simulink model "M_FLCC"  (R2022a)
settings: Solver=ode4  StartTime=0.0  StopTime=100  FixedStep=0.01  RelTol=1e-3
PreLoadFcn:
  | load('BUS_STRUCTURE_FLCC.mat');
InitFcn:
  | load('BUS_STRUCTURE_FLCC.mat');
undefined symbols (not defined in the file or in its folder): f16data
libraries: sharedtransform x6, simulink_extras x4, aerolibatmos2 x1
(part 1 of 2)
settings Model: Creator=ASCL  LastModifiedBy=ASCL
settings DataIOCC: SaveOutput=off  SignalLogging=off  DSMLogging=off  SaveTime=off  ReturnWorkspaceOutputs=off
settings OptimizationCC: BlockReduction=off  DefaultParameterBehavior=Inlined  UseDivisionForNetSlopeComputation=on  GainParamInheritBuiltInType=on  UseFloatMulNetSlope=on  ExpressionFolding=off  PassReuseOutputArgsAs=Individual arguments  ZeroExternalMemoryAtStartup=off  ZeroInternalMemoryAtStartup=off  EfficientFloat2IntCast=on  LifeSpan=inf  OptimizeBlockOrder=speed  DifferentSizesBufferReuse=on  EfficientTunableParamExpr=on
settings DebuggingCC: SignalInfNanChecking=warning  ReadBeforeWriteMsg=EnableAllAsError  WriteAfterWriteMsg=EnableAllAsError  WriteAfterReadMsg=EnableAllAsError  IntegerOverflowMsg=error  ParameterTunabilityLossMsg=error  UniqueDataStoreMsg=error  AssertControl=DisableAll  NonBusSignalsTreatedAsBus=error  SFInvalidInputDataAccessInChartInitDiag=error  SFTransitionOutsideNaturalParentDiag=error  SFUnreachableExecutionPathDiag=error  SFUndirectedBroadcastEventsDiag=error  IntegerSaturationMsg=error
settings HardwareCC: ProdBitPerPointer=32  ProdBitPerSizeT=32  ProdBitPerPtrDiffT=32  ProdLargestAtomicInteger=Long  ProdLargestAtomicFloat=Double  ProdEndianess=BigEndian  ProdWordSize=32  ProdLongLongMode=on  ProdHWDeviceType=Freescale->MPC83xx
settings ModelReferenceCC: ModelReferenceNumInstancesAllowed=Single
settings SFSimCC: SimCustomHeaderCode="#include \"MAP.h\""  SimUserSources=MAP.c  SimUserLibraries=WS2_32.LIB  CompileTimeRecursionLimit=0  EnableRuntimeRecursion=off  MATLABDynamicMemAlloc=off
settings RTWCC: SystemTargetFile=ert.tlc  TemplateMakefile=ert_default_tmf  GenerateReport=on  RTWUseSimCustomCode=on  CustomHeaderCode="#include \"MAP.h\""  CustomSource=MAP.c  CustomLibrary=WS2_32.LIB  BuildConfiguration=Faster Runs  IncludeHyperlinkInReport=on  LaunchReport=on  GenerateTraceInfo=on  GenerateTraceReport=on  GenerateTraceReportSl=on  GenerateTraceReportSf=on  GenerateTraceReportEml=on
settings CodeAppCC: ForceParamTrailComments=on  IgnoreCustomStorageClasses=off  OperatorAnnotations=on  SimulinkDataObjDesc=on  SFDataObjDesc=on  MATLABFcnDesc=on  InsertBlockDesc=on  StateflowObjectComments=on  MATLABSourceComments=on  EnableCustomComments=on  InlinedPrmAccess=Macros  ReqsInCode=on
settings ERTTargetCC: TargetLangStandard=C99 (ISO)  UtilityFuncGeneration=Shared location  GenerateSampleERTMain=on  IncludeMdlTerminateFcn=off  CombineSignalStateStructs=on  SupportAbsoluteTime=off  SupportNonFinite=off  SupportVariableSizeSignals=on  ParenthesesLevel=Standards  CastingMode=Standards  GenerateSharedConstants=off  InlinedParameterPlacement=NonHierarchical  ERTCustomFileTemplate=example_file_process.tlc  RateTransitionBlockCode=Function  PreserveIfCondition=on  ConvertIfToSwitch=off  EnableSignedLeftShifts=off  EnableSignedRightShifts=off

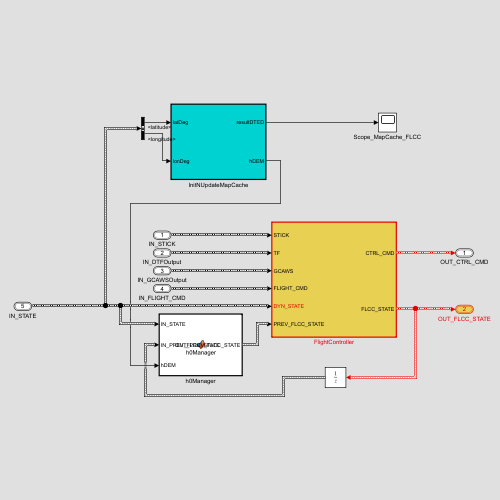
[thumbnail: Simulink's stored preview of the top-level diagram]
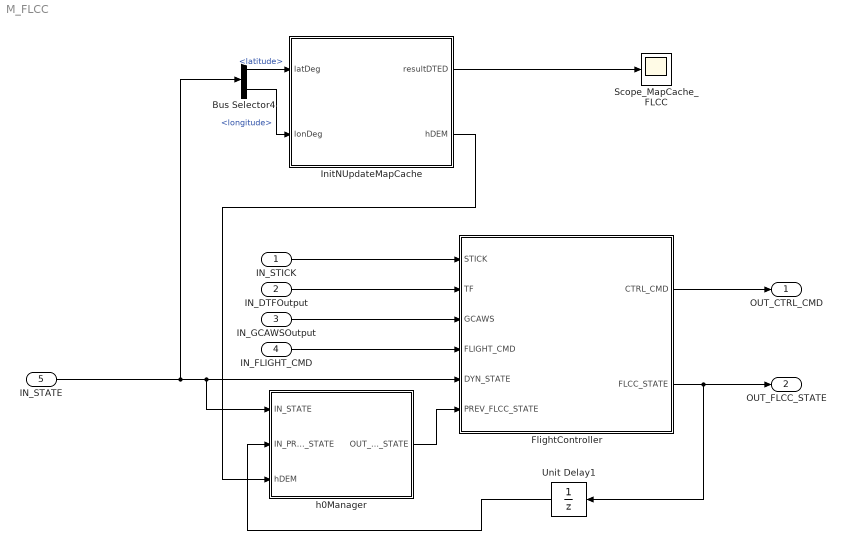
== system M_FLCC ==
  IN_STICK : Inport  OutDataTypeStr=Bus: BUS_FLCC_STICK  Interpolate=off  BusOutputAsStruct=on
  IN_DTFOutput : Inport  Port=2  OutDataTypeStr=Bus: DTFOutput  Interpolate=off  BusOutputAsStruct=on
  IN_GCAWSOutput : Inport  Port=3  OutDataTypeStr=Bus: GCAWSOutput  Interpolate=off  BusOutputAsStruct=on
  IN_FLIGHT_CMD : Inport  Port=4  OutDataTypeStr=Bus: BUS_FLCC_FLIGHT_CMD  Interpolate=off  BusOutputAsStruct=on
  IN_STATE : Inport  Port=5  OutDataTypeStr=Bus: BUS_DYN_STATE  Interpolate=off  BusOutputAsStruct=on
  Bus Selector4 : BusSelector  OutputSignals=latitude,longitude
  FlightController : Subsystem  TreatAsAtomicUnit=on
  InitNUpdateMapCache : Subsystem  TreatAsAtomicUnit=on
  Scope_MapCache_FLCC : Scope
  Unit Delay1 : UnitDelay  SampleTime=0.01  HasFrameUpgradeWarning=on
  h0Manager : MATLAB Function  TreatAsAtomicUnit=on
  OUT_CTRL_CMD : Outport  OutDataTypeStr=Bus: BUS_FLCC_CTRL_CMD  VectorParamsAs1DForOutWhenUnconnected=off  BusOutputAsStruct=on
  OUT_FLCC_STATE : Outport  Port=2  OutDataTypeStr=Bus: BUS_FLCC_AP_STATE  VectorParamsAs1DForOutWhenUnconnected=off  BusOutputAsStruct=on
  wires:
  FlightController/1(CTRL_CMD) -> OUT_CTRL_CMD/1
  IN_STICK/1 -> FlightController/1(STICK)
  IN_STATE/1 -> Bus Selector4/1, h0Manager/1(IN_STATE), FlightController/5(DYN_STATE)
  IN_DTFOutput/1 -> FlightController/2(TF)
  FlightController/2(FLCC_STATE) -> OUT_FLCC_STATE/1, Unit Delay1/1
  IN_GCAWSOutput/1 -> FlightController/3(GCAWS)
  Unit Delay1/1 -> h0Manager/2(IN_PREV_FLCC_STATE)
  Bus Selector4/1 -> InitNUpdateMapCache/1(latDeg)  "<latitude>"
  Bus Selector4/2 -> InitNUpdateMapCache/2(lonDeg)  "<longitude>"
  InitNUpdateMapCache/1(resultDTED) -> Scope_MapCache_FLCC/1
  h0Manager/1(OUT_PREV_FLCC_STATE) -> FlightController/6(PREV_FLCC_STATE)
  InitNUpdateMapCache/2(hDEM) -> h0Manager/3(hDEM)
  IN_FLIGHT_CMD/1 -> FlightController/4(FLIGHT_CMD)

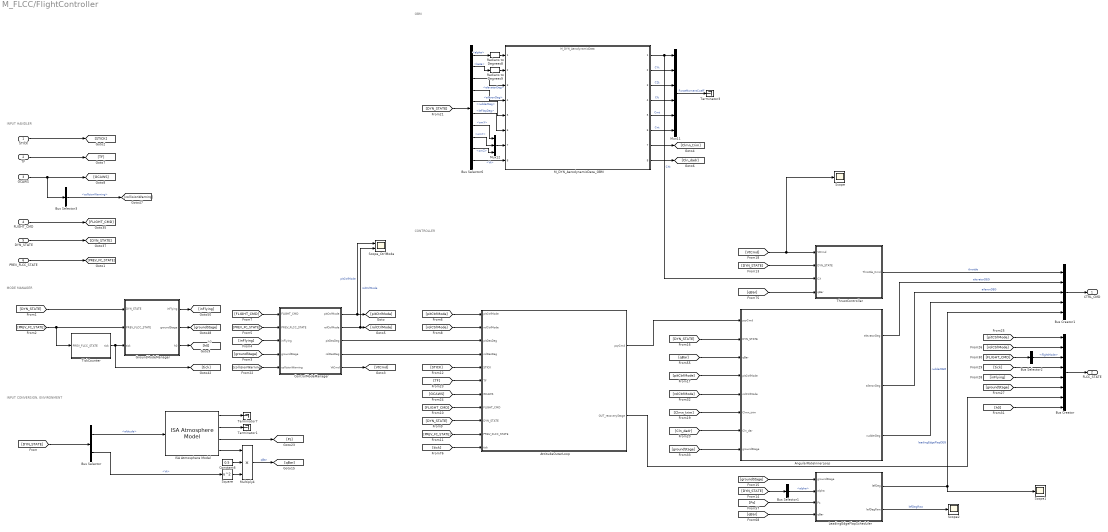
== system M_FLCC/FlightController ==
  note: h0
  note: OBM
  note: CONTROLLER
  note: MODE MANAGER
  note: INPUT CONVERSION, ENVIRONMENT
  note: INPUT HANDLER
  STICK : Inport  OutDataTypeStr=Bus: BUS_FLCC_STICK
  TF : Inport  Port=2  OutDataTypeStr=Bus: DTFOutput
  GCAWS : Inport  Port=3  OutDataTypeStr=Bus: GCAWSOutput
  FLIGHT_CMD : Inport  Port=4  OutDataTypeStr=Bus: BUS_FLCC_FLIGHT_CMD
  DYN_STATE : Inport  Port=5  OutDataTypeStr=Bus: BUS_DYN_STATE
  PREV_FLCC_STATE : Inport  Port=6  OutDataTypeStr=Bus: BUS_FLCC_AP_STATE
  AngularRateInnerLoop : Subsystem
  AttitudeOuterLoop : Subsystem
  Bus Creator : BusCreator  Inputs=8  OutDataTypeStr=Bus: BUS_FLCC_AP_STATE  NonVirtualBus=on
      settings: InheritFromInputs=off
  Bus Creator1 : BusCreator  Inputs=5  OutDataTypeStr=Bus: BUS_FLCC_CTRL_CMD  NonVirtualBus=on
      settings: InheritFromInputs=off
  Bus Selector : BusSelector  OutputSignals=altitude,Vt
  Bus Selector1 : BusSelector  OutputSignals=alpha
  Bus Selector2 : BusSelector  OutputSignals=flightMode
  Bus Selector3 : BusSelector  OutputSignals=collisionWarning
  Bus Selector6 : BusSelector  OutputSignals=alpha,beta,elevatorDeg,aileronDeg,rudderDeg,leFlapDeg,omX,omY,omZ,Vt
  Constant6 : Constant  Value=0.5
  ControlModeManager : MATLAB Function  TreatAsAtomicUnit=on
  GroundModeManager : MATLAB Function  TreatAsAtomicUnit=on
  ISA Atmosphere Model : aerolibatmos2/ISA Atmosphere Model  custom=off  g=9.80665  gamma=1.4  R=287.0531  L=0.0065  h_trop=11000  h_strat=20000  rho0=1.225  P0=101325  T0=288.15  h0=0
  LeadingEdgeFlapScheduler : MATLAB Function  TreatAsAtomicUnit=on
  M_DYN_AerodynamicData_OBM : ModelReference  ModelNameDialog=M_DYN_AerodynamicData.slx  SimulationMode=Normal  ModelReferenceVersion=1.97
  Multiply4 : Product  Inputs=3
  Mux11 : Mux  Inputs=6
  Mux12 : Mux  Inputs=3
  Radians to Degrees8 : simulink_extras/Transformations/Radians to Degrees
  Radians to Degrees9 : simulink_extras/Transformations/Radians to Degrees
  Scope : Scope
  Scope1 : Scope
  Scope2 : Scope
  Scope_CtrlMode : Scope  NumInputPorts=2
  Square : Math  Operator=square  SignedPower=on
  Terminator1 : Terminator
  Terminator3 : Terminator
  Terminator7 : Terminator
  ThrustController : Subsystem
  TickCounter : MATLAB Function  TreatAsAtomicUnit=on
  CTRL_CMD : Outport  OutDataTypeStr=Bus: BUS_FLCC_CTRL_CMD  VectorParamsAs1DForOutWhenUnconnected=off
  FLCC_STATE : Outport  Port=2  OutDataTypeStr=Bus: BUS_FLCC_AP_STATE  VectorParamsAs1DForOutWhenUnconnected=off
  wires:
  DYN_STATE/1 -> [DYN_STATE]
  ISA Atmosphere Model/1 -> Terminator7/1
  ISA Atmosphere Model/2 -> Terminator1/1
  ISA Atmosphere Model/3 -> [Ps]
  ISA Atmosphere Model/4 -> Multiply4/1
  Constant6/1 -> Multiply4/2
  Square/1 -> Multiply4/3
  Multiply4/1 -> [qBar]  "qBar"
  LeadingEdgeFlapScheduler/1(lefDeg) -> Scope1/1, Bus Creator1/5  "leadingEdgeFlapDEG"
  Bus Creator/1 -> FLCC_STATE/1
  [pitCtrlMode] -> Bus Creator/1
  [rolCtrlMode] -> Bus Creator/2
  Bus Selector3/1 -> [collisionWarning]  "<collisionWarning>"
  TickCounter/1(tick) -> [tick], GroundModeManager/3(tick)
  GroundModeManager/1(inFlying) -> [inFlying]
  ControlModeManager/2(rolCtrlMode) -> Scope_CtrlMode/2, [rolCtrlMode]  "rolCtrlMode"
  ControlModeManager/1(pitCtrlMode) -> Scope_CtrlMode/1, [pitCtrlMode]  "pitCtrlMode"
  [Ps] -> LeadingEdgeFlapScheduler/3(Ps)
  [qBar] -> LeadingEdgeFlapScheduler/4(qBar)
  GroundModeManager/2(groundStage) -> [groundStage]
  STICK/1 -> [STICK]
  AttitudeOuterLoop/1(pqrCmd) -> AngularRateInnerLoop/1(pqrCmd)
  M_DYN_AerodynamicData_OBM/6 -> Mux11/6  "Cnt"
  M_DYN_AerodynamicData_OBM/5 -> Mux11/5  "Cmt"
  M_DYN_AerodynamicData_OBM/4 -> Mux11/4  "Clt"
  M_DYN_AerodynamicData_OBM/2 -> Mux11/2  "CYt"
  M_DYN_AerodynamicData_OBM/1 -> Mux11/1, ThrustController/3(CX)  "CXt"
  M_DYN_AerodynamicData_OBM/3 -> Mux11/3  "CZt"
  Mux11/1 -> Terminator3/1  "ForceMomentCoeff"
  [qBar] -> AngularRateInnerLoop/3(qBar)
  [qBar] -> ThrustController/4(qBar)
  ThrustController/1(Throttle_Cmd) -> Bus Creator1/1  "throttle"
  Bus Selector6/10 -> M_DYN_AerodynamicData_OBM/8  "<Vt>"
  Bus Selector6/1 -> Radians to Degrees8/1  "<alpha>"
  Bus Selector6/2 -> Radians to Degrees9/1  "<beta>"
  Radians to Degrees8/1 -> M_DYN_AerodynamicData_OBM/1
  Radians to Degrees9/1 -> M_DYN_AerodynamicData_OBM/2
  Bus Selector6/3 -> M_DYN_AerodynamicData_OBM/3  "<elevatorDeg>"
  Bus Selector6/4 -> M_DYN_AerodynamicData_OBM/4  "<aileronDeg>"
  Bus Selector6/5 -> M_DYN_AerodynamicData_OBM/5  "<rudderDeg>"
  Bus Selector6/6 -> M_DYN_AerodynamicData_OBM/6  "<leFlapDeg>"
  Mux12/1 -> M_DYN_AerodynamicData_OBM/7
  Bus Selector6/9 -> Mux12/3  "<omZ>"
  Bus Selector6/8 -> Mux12/2  "<omY>"
  Bus Selector6/7 -> Mux12/1  "<omX>"
  [tick] -> AttitudeOuterLoop/11(tick)
  ControlModeManager/3(pitDesDeg) -> AttitudeOuterLoop/3(pitDesDeg)
  ControlModeManager/4(rolDesDeg) -> AttitudeOuterLoop/4(rolDesDeg)
  [DYN_STATE] -> Bus Selector/1
  [DYN_STATE] -> GroundModeManager/1(DYN_STATE)
  PREV_FLCC_STATE/1 -> [PREV_FC_STATE]
  [PREV_FC_STATE] -> TickCounter/1(PREV_FLCC_STATE), GroundModeManager/2(PREV_FLCC_STATE)
  [groundStage] -> ControlModeManager/4(groundStage)
  [inFlying] -> ControlModeManager/3(inFlying)
  [PREV_FC_STATE] -> ControlModeManager/2(PREV_FLCC_STATE)
  [FLIGHT_CMD] -> ControlModeManager/1(FLIGHT_CMD)
  Bus Selector/1 -> ISA Atmosphere Model/1  "<altitude>"
  Bus Selector/2 -> Square/1  "<Vt>"
  [DYN_STATE] -> AttitudeOuterLoop/9(DYN_STATE)
  [FLIGHT_CMD] -> AttitudeOuterLoop/8(FLIGHT_CMD)
  [PREV_FC_STATE] -> AttitudeOuterLoop/10(PREV_FLCC_STATE)
  [STICK] -> AttitudeOuterLoop/5(STICK)
  [DYN_STATE] -> ThrustController/2(DYN_STATE)
  [DYN_STATE] -> Bus Selector1/1
  Bus Selector1/1 -> LeadingEdgeFlapScheduler/2(alpha)  "<alpha>"
  [groundStage] -> LeadingEdgeFlapScheduler/1(groundStage)
  [DYN_STATE] -> AngularRateInnerLoop/2(DYN_STATE)
  Bus Creator1/1 -> CTRL_CMD/1
  AngularRateInnerLoop/1(elevatorDeg) -> Bus Creator1/2  "elevatorDEG"
  AngularRateInnerLoop/2(aileronDeg) -> Bus Creator1/3  "aileronDEG"
  AngularRateInnerLoop/3(rudderDeg) -> Bus Creator1/4  "rudderDEG"
  ControlModeManager/5(VtCmd) -> [VtCmd]
  [VtCmd] -> Scope/1, ThrustController/1(VtCmd)
  M_DYN_AerodynamicData_OBM/8 -> [Cln_dadr]
  M_DYN_AerodynamicData_OBM/7 -> [Clmn_trim]
  [Clmn_trim] -> AngularRateInnerLoop/6(Clmn_trim)
  [Cln_dadr] -> AngularRateInnerLoop/7(Cln_dar)
  [DYN_STATE] -> Bus Selector6/1
  [collisionWarning] -> ControlModeManager/5(collisionWarning)
  GCAWS/1 -> Bus Selector3/1, [GCAWS]
  TF/1 -> [TF]
  [GCAWS] -> AttitudeOuterLoop/7(GCAWS)
  [TF] -> AttitudeOuterLoop/6(TF)
  [rolCtrlMode] -> AttitudeOuterLoop/2(rolCtrlMode)
  [pitCtrlMode] -> AttitudeOuterLoop/1(pitCtrlMode)
  [groundStage] -> Bus Creator/6
  [inFlying] -> Bus Creator/5
  [tick] -> Bus Creator/4
  AttitudeOuterLoop/2(OUT_recoveryStage) -> Bus Creator/7
  [FLIGHT_CMD] -> Bus Selector2/1
  Bus Selector2/1 -> Bus Creator/3  "<flightMode>"
  GroundModeManager/3(h0) -> [h0]
  [h0] -> Bus Creator/8
  [pitCtrlMode] -> AngularRateInnerLoop/4(pitCtrlMode)
  [rolCtrlMode] -> AngularRateInnerLoop/5(rolCtrlMode)
  [groundStage] -> AngularRateInnerLoop/8(groundStage)
  LeadingEdgeFlapScheduler/2(lefDegRaw) -> Scope2/1  "lefDegRaw"
  FLIGHT_CMD/1 -> [FLIGHT_CMD]

== system M_FLCC/InitNUpdateMapCache ==
  latDeg : Inport  OutDataTypeStr=double
  lonDeg : Inport  Port=2  OutDataTypeStr=double
  If : If  NumInputs=2  IfExpression=(u1 == 0)  ShowElse=off
  InitializeMAP : MATLAB Function  TreatAsAtomicUnit=on  SystemSampleTime=0.01
  UpdateCache : Subsystem  TreatAsAtomicUnit=on
  resultDTED : Outport  VectorParamsAs1DForOutWhenUnconnected=off
  hDEM : Outport  Port=2
  wires:
  lonDeg/1 -> InitializeMAP/2(lonDeg), UpdateCache/2(lon)
  UpdateCache/1(result) -> resultDTED/1
  InitializeMAP/1(successDTED) -> If/1
  latDeg/1 -> InitializeMAP/1(latDeg), UpdateCache/1(lat)
  InitializeMAP/2(successDVOF) -> If/2
  If/1 -> UpdateCache/Action
  UpdateCache/2(hDEM) -> hDEM/1

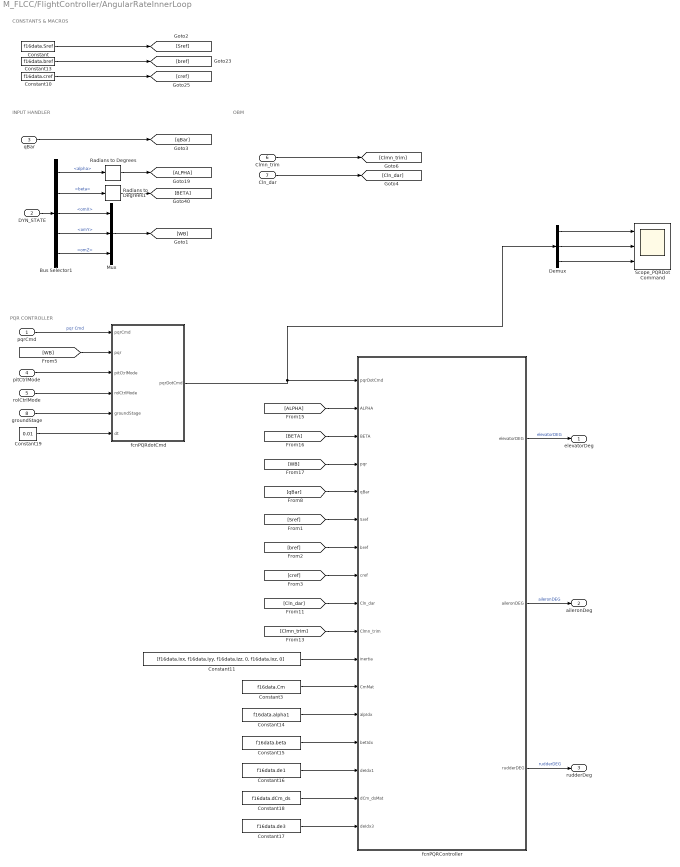
== system M_FLCC/FlightController/AngularRateInnerLoop ==
  note: PQR CONTROLLER
  note: INPUT HANDLER
  note: OBM
  note: CONSTANTS & MACROS
  pqrCmd : Inport
  DYN_STATE : Inport  Port=2
  qBar : Inport  Port=3
  pitCtrlMode : Inport  Port=4
  rolCtrlMode : Inport  Port=5
  Clmn_trim : Inport  Port=6
  Cln_dar : Inport  Port=7
  groundStage : Inport  Port=8
  Bus Selector1 : BusSelector  OutputSignals=alpha,beta,omX,omY,omZ
  Constant : Constant  Value=f16data.Sref
  Constant10 : Constant  Value=f16data.cref
  Constant11 : Constant  Value=[f16data.Ixx, f16data.Iyy, f16data.Izz, 0, f16data.Ixz, 0]
  Constant13 : Constant  Value=f16data.bref
  Constant14 : Constant  Value=f16data.alpha1
  Constant15 : Constant  Value=f16data.beta
  Constant16 : Constant  Value=f16data.de1
  Constant17 : Constant  Value=f16data.de3
  Constant18 : Constant  Value=f16data.dCm_ds
  Constant19 : Constant  Value=0.01
  Constant3 : Constant  Value=f16data.Cm
  Demux : Demux  Outputs=3
  Mux : Mux  Inputs=3
  Radians to Degrees : simulink_extras/Transformations/Radians to Degrees
  Radians to Degrees1 : simulink_extras/Transformations/Radians to Degrees
  Scope_PQRDot Command : Scope  NumInputPorts=3
  fcnPQRController : MATLAB Function  TreatAsAtomicUnit=on
  fcnPQRdotCmd : MATLAB Function  TreatAsAtomicUnit=on  SystemSampleTime=0.01
  elevatorDeg : Outport
  aileronDeg : Outport  Port=2
  rudderDeg : Outport  Port=3
  wires:
  Bus Selector1/1 -> Radians to Degrees/1  "<alpha>"
  Mux/1 -> [WB]
  Bus Selector1/2 -> Radians to Degrees1/1  "<beta>"
  [WB] -> fcnPQRdotCmd/2(pqr)
  pqrCmd/1 -> fcnPQRdotCmd/1(pqrCmd)  "pqr Cmd"
  Constant11/1 -> fcnPQRController/11(inertia)
  [qBar] -> fcnPQRController/5(qBar)
  qBar/1 -> [qBar]
  [Sref] -> fcnPQRController/6(Sref)
  [bref] -> fcnPQRController/7(bref)
  [cref] -> fcnPQRController/8(cref)
  [Cln_dar] -> fcnPQRController/9(Cln_dar)
  Constant3/1 -> fcnPQRController/12(CmMat)
  Constant14/1 -> fcnPQRController/13(alpIdx)
  Constant15/1 -> fcnPQRController/14(betIdx)
  Constant16/1 -> fcnPQRController/15(deIdx1)
  Constant18/1 -> fcnPQRController/16(dCm_dsMat)
  Constant17/1 -> fcnPQRController/17(deIdx3)
  [ALPHA] -> fcnPQRController/2(ALPHA)
  [BETA] -> fcnPQRController/3(BETA)
  fcnPQRController/1(elevatorDEG) -> elevatorDeg/1  "elevatorDEG"
  fcnPQRController/3(rudderDEG) -> rudderDeg/1  "rudderDEG"
  [WB] -> fcnPQRController/4(pqr)
  [Clmn_trim] -> fcnPQRController/10(Clmn_trim)
  Constant19/1 -> fcnPQRdotCmd/6(dt)
  Clmn_trim/1 -> [Clmn_trim]
  Cln_dar/1 -> [Cln_dar]
  Constant/1 -> [Sref]
  Constant10/1 -> [cref]
  Constant13/1 -> [bref]
  fcnPQRdotCmd/1(pqrDotCmd) -> Demux/1, fcnPQRController/1(pqrDotCmd)
  DYN_STATE/1 -> Bus Selector1/1
  Bus Selector1/3 -> Mux/1  "<omX>"
  Bus Selector1/4 -> Mux/2  "<omY>"
  Bus Selector1/5 -> Mux/3  "<omZ>"
  Radians to Degrees/1 -> [ALPHA]
  Radians to Degrees1/1 -> [BETA]
  fcnPQRController/2(aileronDEG) -> aileronDeg/1  "aileronDEG"
  Demux/3 -> Scope_PQRDot Command/3
  Demux/1 -> Scope_PQRDot Command/1
  Demux/2 -> Scope_PQRDot Command/2
  pitCtrlMode/1 -> fcnPQRdotCmd/3(pitCtrlMode)
  rolCtrlMode/1 -> fcnPQRdotCmd/4(rolCtrlMode)
  groundStage/1 -> fcnPQRdotCmd/5(groundStage)

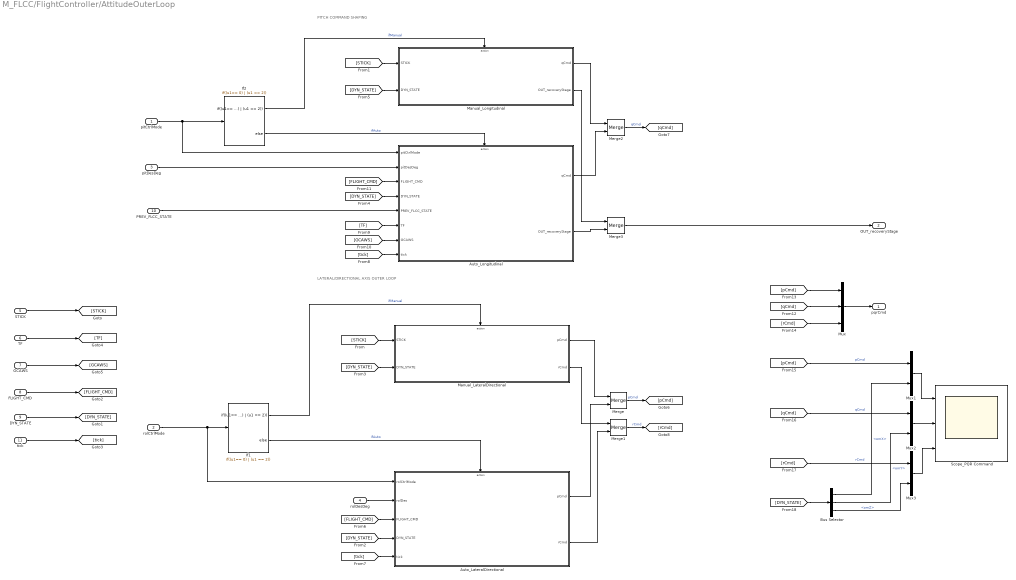
== system M_FLCC/FlightController/AttitudeOuterLoop ==
  note: PITCH COMMAND SHAPING
  note: LATERAL/DIRECTIONAL AXIS OUTER LOOP
  pitCtrlMode : Inport
  rolCtrlMode : Inport  Port=2
  pitDesDeg : Inport  Port=3
  rolDesDeg : Inport  Port=4
  STICK : Inport  Port=5
  TF : Inport  Port=6
  GCAWS : Inport  Port=7
  FLIGHT_CMD : Inport  Port=8
  DYN_STATE : Inport  Port=9
  PREV_FLCC_STATE : Inport  Port=10
  tick : Inport  Port=11
  Auto_LateralDirectional : Subsystem  TreatAsAtomicUnit=on
  Auto_Longitudinal : Subsystem  TreatAsAtomicUnit=on
  Bus Selector : BusSelector  OutputSignals=omX,omY,omZ
  If1 : If  IfExpression=(u1== 0) | (u1 == 2)
  If2 : If  IfExpression=(u1== 0) | (u1 == 2)
  Manual_LateralDirectional : Subsystem  TreatAsAtomicUnit=on
  Manual_Longitudinal : Subsystem  TreatAsAtomicUnit=on
  Merge{,1..3} (4 alike) : Merge
  Mux : Mux  Inputs=3
  Mux1 : Mux  Inputs=2
  Mux2 : Mux  Inputs=2
  Mux3 : Mux  Inputs=2
  Scope_PQR Command : Scope  NumInputPorts=3
  pqrCmd : Outport
  OUT_recoveryStage : Outport  Port=2
  wires:
  rolDesDeg/1 -> Auto_LateralDirectional/2(rolDes)
  rolCtrlMode/1 -> Auto_LateralDirectional/1(rolCtrlMode), If1/1
  If1/1 -> Manual_LateralDirectional/Action  "ifManual"
  If1/2 -> Auto_LateralDirectional/Action  "ifAuto"
  Manual_LateralDirectional/1(pCmd) -> Merge/1
  Auto_LateralDirectional/1(pCmd) -> Merge/2
  Manual_LateralDirectional/2(rCmd) -> Merge1/1
  Auto_LateralDirectional/2(rCmd) -> Merge1/2
  Mux/1 -> pqrCmd/1
  Merge/1 -> [pCmd]  "pCmd"
  Merge1/1 -> [rCmd]  "rCmd"
  pitCtrlMode/1 -> Auto_Longitudinal/1(pitCtrlMode), If2/1
  If2/1 -> Manual_Longitudinal/Action  "ifManual"
  Manual_Longitudinal/1(qCmd) -> Merge2/1
  Merge2/1 -> [qCmd]  "qCmd"
  Auto_Longitudinal/1(qCmd) -> Merge2/2
  pitDesDeg/1 -> Auto_Longitudinal/2(pitDesDeg)
  If2/2 -> Auto_Longitudinal/Action  "ifAuto"
  PREV_FLCC_STATE/1 -> Auto_Longitudinal/5(PREV_FLCC_STATE)
  STICK/1 -> [STICK]
  [STICK] -> Manual_LateralDirectional/1(STICK)
  [STICK] -> Manual_Longitudinal/1(STICK)
  DYN_STATE/1 -> [DYN_STATE]
  [DYN_STATE] -> Auto_LateralDirectional/4(DYN_STATE)
  [DYN_STATE] -> Auto_Longitudinal/4(DYN_STATE)
  [DYN_STATE] -> Manual_Longitudinal/2(DYN_STATE)
  [DYN_STATE] -> Manual_LateralDirectional/2(DYN_STATE)
  FLIGHT_CMD/1 -> [FLIGHT_CMD]
  [FLIGHT_CMD] -> Auto_LateralDirectional/3(FLIGHT_CMD)
  [tick] -> Auto_LateralDirectional/5(tick)
  [tick] -> Auto_Longitudinal/8(tick)
  tick/1 -> [tick]
  TF/1 -> [TF]
  GCAWS/1 -> [GCAWS]
  [TF] -> Auto_Longitudinal/6(TF)
  [GCAWS] -> Auto_Longitudinal/7(GCAWS)
  [FLIGHT_CMD] -> Auto_Longitudinal/3(FLIGHT_CMD)
  Auto_Longitudinal/2(OUT_recoveryStage) -> Merge3/2
  Manual_Longitudinal/2(OUT_recoveryStage) -> Merge3/1
  Merge3/1 -> OUT_recoveryStage/1
  Mux1/1 -> Scope_PQR Command/1
  [qCmd] -> Mux/2
  [pCmd] -> Mux/1
  [rCmd] -> Mux/3
  Mux2/1 -> Scope_PQR Command/2
  Mux3/1 -> Scope_PQR Command/3
  [pCmd] -> Mux1/1  "pCmd"
  [qCmd] -> Mux2/1  "qCmd"
  [rCmd] -> Mux3/1  "rCmd"
  [DYN_STATE] -> Bus Selector/1
  Bus Selector/1 -> Mux1/2  "<omX>"
  Bus Selector/2 -> Mux2/2  "<omY>"
  Bus Selector/3 -> Mux3/2  "<omZ>"

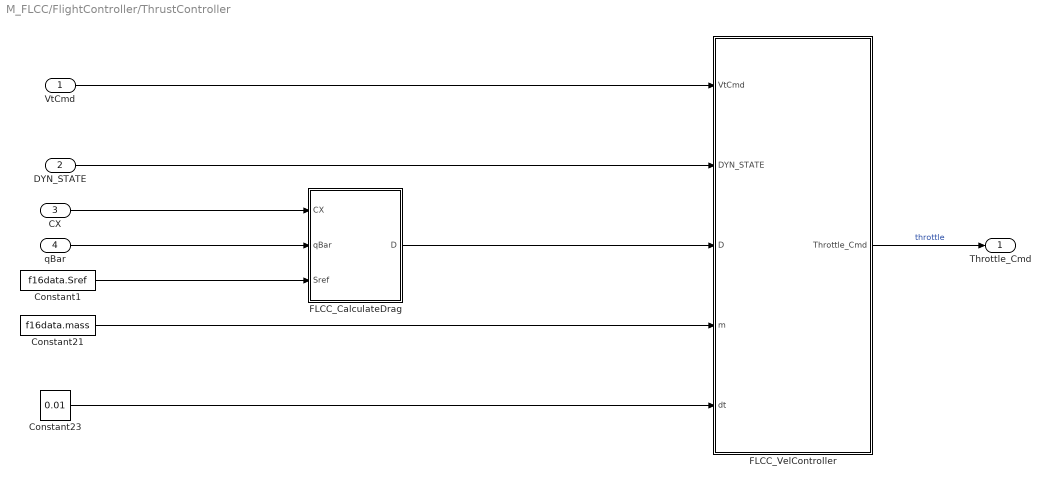
== system M_FLCC/FlightController/ThrustController ==
  VtCmd : Inport
  DYN_STATE : Inport  Port=2
  CX : Inport  Port=3
  qBar : Inport  Port=4
  Constant1 : Constant  Value=f16data.Sref
  Constant21 : Constant  Value=f16data.mass
  Constant23 : Constant  Value=0.01
  FLCC_CalculateDrag : MATLAB Function  TreatAsAtomicUnit=on
  FLCC_VelController : MATLAB Function  TreatAsAtomicUnit=on  SystemSampleTime=0.01
  Throttle_Cmd : Outport
  wires:
  Constant21/1 -> FLCC_VelController/4(m)
  VtCmd/1 -> FLCC_VelController/1(VtCmd)
  DYN_STATE/1 -> FLCC_VelController/2(DYN_STATE)
  FLCC_CalculateDrag/1(D) -> FLCC_VelController/3(D)
  Constant23/1 -> FLCC_VelController/5(dt)
  FLCC_VelController/1(Throttle_Cmd) -> Throttle_Cmd/1  "throttle"
  CX/1 -> FLCC_CalculateDrag/1(CX)
  Constant1/1 -> FLCC_CalculateDrag/3(Sref)
  qBar/1 -> FLCC_CalculateDrag/2(qBar)

== system M_FLCC/InitNUpdateMapCache/UpdateCache ==
  lat : Inport
  lon : Inport  Port=2
  Action Port : ActionPort  ActionPortLabel=if((u1 == 0))
  UpdateCache : MATLAB Function  TreatAsAtomicUnit=on  SystemSampleTime=0.01
  result : Outport  VectorParamsAs1DForOutWhenUnconnected=off
  hDEM : Outport  Port=2
  wires:
  UpdateCache/1(result) -> result/1
  lat/1 -> UpdateCache/1(lat)
  lon/1 -> UpdateCache/2(lon)
  UpdateCache/2(hDEM) -> hDEM/1

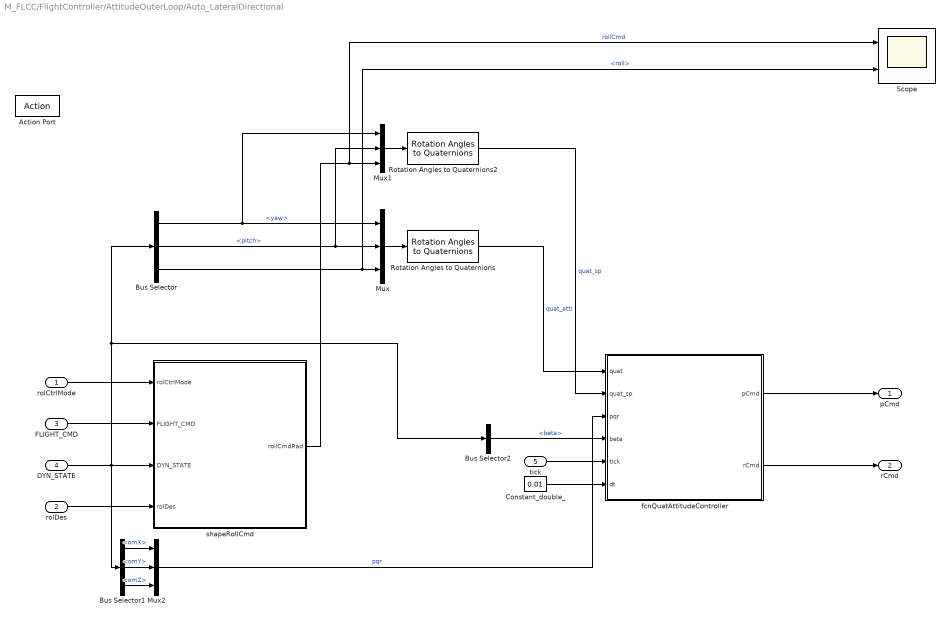
== system M_FLCC/FlightController/AttitudeOuterLoop/Auto_LateralDirectional ==
  rolCtrlMode : Inport
  rolDes : Inport  Port=2
  FLIGHT_CMD : Inport  Port=3  OutDataTypeStr=Bus: BUS_FLCC_FLIGHT_CMD
  DYN_STATE : Inport  Port=4  OutDataTypeStr=Bus: BUS_DYN_STATE
  tick : Inport  Port=5
  Action Port : ActionPort  ActionPortLabel=else
  Bus Selector : BusSelector  OutputSignals=yaw,pitch,roll
  Bus Selector1 : BusSelector  OutputSignals=omX,omY,omZ
  Bus Selector2 : BusSelector  OutputSignals=beta
  Constant_double_ : Constant  Value=0.01  OutDataTypeStr=double
  Mux : Mux  Inputs=3
  Mux1 : Mux  Inputs=3
  Mux2 : Mux  Inputs=3
  Rotation Angles to Quaternions : sharedtransform/Rotation Angles to Quaternions  rotationOrder=ZYX  aMode=aMode
      settings: SourceProductBaseCode=AE,PW,DR,MT,VE
  Rotation Angles to Quaternions2 : sharedtransform/Rotation Angles to Quaternions  rotationOrder=ZYX  aMode=aMode
      settings: SourceProductBaseCode=AE,PW,DR,MT,VE
  Scope : Scope  NumInputPorts=2
  fcnQuatAttitudeController : MATLAB Function  TreatAsAtomicUnit=on
  shapeRollCmd : MATLAB Function  TreatAsAtomicUnit=on
  pCmd : Outport
  rCmd : Outport  Port=2
  wires:
  rolCtrlMode/1 -> shapeRollCmd/1(rolCtrlMode)
  FLIGHT_CMD/1 -> shapeRollCmd/2(FLIGHT_CMD)
  DYN_STATE/1 -> Bus Selector/1, Bus Selector2/1, Bus Selector1/1, shapeRollCmd/3(DYN_STATE)
  Mux/1 -> Rotation Angles to Quaternions/1
  Constant_double_/1 -> fcnQuatAttitudeController/6(dt)
  Bus Selector/2 -> Mux/2, Mux1/2  "<pitch>"
  Bus Selector/1 -> Mux/1, Mux1/1  "<yaw>"
  Bus Selector/3 -> Scope/2, Mux/3  "<roll>"
  Rotation Angles to Quaternions/1 -> fcnQuatAttitudeController/1(quat)  "quat_atti"
  shapeRollCmd/1(rollCmdRad) -> Scope/1, Mux1/3  "rollCmd"
  Mux1/1 -> Rotation Angles to Quaternions2/1
  Rotation Angles to Quaternions2/1 -> fcnQuatAttitudeController/2(quat_sp)  "quat_sp"
  Mux2/1 -> fcnQuatAttitudeController/3(pqr)  "pqr"
  Bus Selector1/1 -> Mux2/1  "<omX>"
  Bus Selector1/2 -> Mux2/2  "<omY>"
  Bus Selector1/3 -> Mux2/3  "<omZ>"
  fcnQuatAttitudeController/2(rCmd) -> rCmd/1
  fcnQuatAttitudeController/1(pCmd) -> pCmd/1
  rolDes/1 -> shapeRollCmd/4(rolDes)
  tick/1 -> fcnQuatAttitudeController/5(tick)
  Bus Selector2/1 -> fcnQuatAttitudeController/4(beta)  "<beta>"

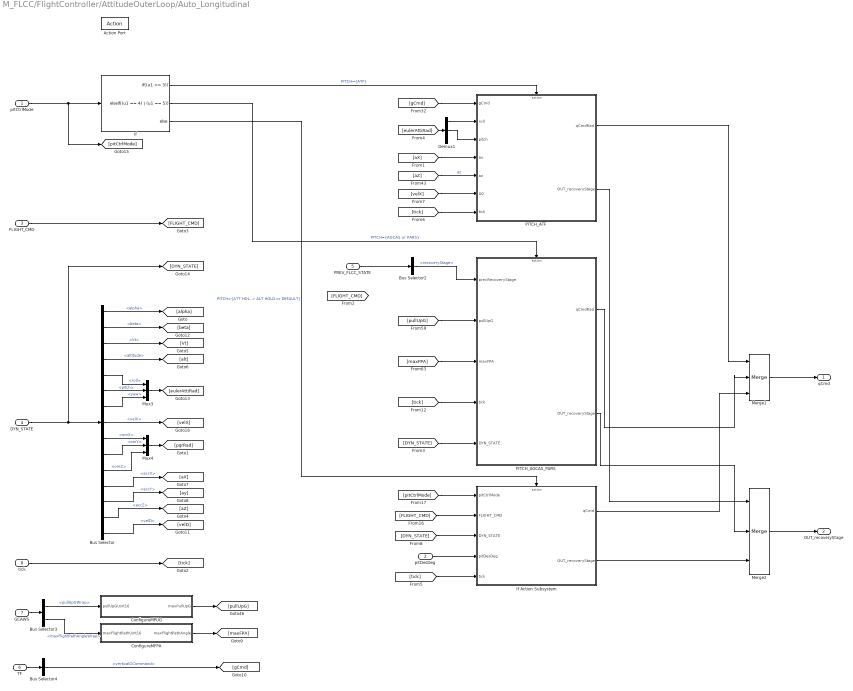
== system M_FLCC/FlightController/AttitudeOuterLoop/Auto_Longitudinal ==
  pitCtrlMode : Inport
  pitDesDeg : Inport  Port=2
  FLIGHT_CMD : Inport  Port=3
  DYN_STATE : Inport  Port=4
  PREV_FLCC_STATE : Inport  Port=5
  TF : Inport  Port=6
  GCAWS : Inport  Port=7
  tick : Inport  Port=8
  Action Port : ActionPort  ActionPortLabel=else
  Bus Selector : BusSelector  OutputSignals=alpha,beta,Vt,altitude,roll,pitch,yaw,velX,omX,omY,omZ,accX,accY,accZ,velD
  Bus Selector2 : BusSelector  OutputSignals=recoveryStage
  Bus Selector3 : BusSelector  OutputSignals=pullUpGWrap,maxFlightPathAngleWrap
  Bus Selector4 : BusSelector  OutputSignals=verticalGCommand
  ConfigureMFPA : MATLAB Function  TreatAsAtomicUnit=on
      settings: RTWSystemCode=Nonreusable function  RTWFcnNameOpts=Use subsystem name  FunctionInterfaceSpec=Allow arguments (Match graphical interface)
  ConfigureMPUG : MATLAB Function  TreatAsAtomicUnit=on
      settings: RTWSystemCode=Nonreusable function  RTWFcnNameOpts=Use subsystem name  FunctionInterfaceSpec=Allow arguments (Match graphical interface)
  Demux1 : Demux  Outputs=3
  If : If  IfExpression=(u1 == 3)  ElseIfExpressions=(u1 == 4) | (u1 == 5)
  If Action Subsystem : Subsystem  TreatAsAtomicUnit=on
  Merge1 : Merge  Inputs=3
  Merge2 : Merge  Inputs=3
  Mux3 : Mux  Inputs=3
  Mux4 : Mux  Inputs=3
  PITCH_AGCAS_PARS : Subsystem  TreatAsAtomicUnit=on
  PITCH_ATF : Subsystem  TreatAsAtomicUnit=on
  qCmd : Outport
  OUT_recoveryStage : Outport  Port=2
  wires:
  [aZ] -> PITCH_ATF/5(az)  "az"
  [maxFPA] -> PITCH_AGCAS_PARS/3(maxFPA)
  Bus Selector2/1 -> PITCH_AGCAS_PARS/1(prevRecoveryStage)  "<recoveryStage>"
  If/1 -> PITCH_ATF/Action  "PITCH={ATF}"
  [pullUpG] -> PITCH_AGCAS_PARS/2(pullUpG)
  [velX] -> PITCH_ATF/6(U0)
  [aX] -> PITCH_ATF/4(ax)
  [gCmd] -> PITCH_ATF/1(gCmd)
  If/2 -> PITCH_AGCAS_PARS/Action  "PITCH={AGCAS or PARS}"
  pitCtrlMode/1 -> [pitCtrlMode], If/1
  DYN_STATE/1 -> [DYN_STATE], Bus Selector/1
  Bus Selector/1 -> [alpha]  "<alpha>"
  Bus Selector/5 -> Mux3/1  "<roll>"
  If/3 -> If Action Subsystem/Action  "PITCH={ATT HOLD or ALT HOLD or DEFAULT}"
  FLIGHT_CMD/1 -> [FLIGHT_CMD]
  Bus Selector/3 -> [Vt]  "<Vt>"
  Bus Selector/4 -> [alt]  "<altitude>"
  Bus Selector/14 -> [aZ]  "<accZ>"
  Bus Selector/12 -> [aX]  "<accX>"
  Bus Selector/10 -> Mux4/2  "<omY>"
  Bus Selector/7 -> Mux3/3  "<yaw>"
  Bus Selector/9 -> Mux4/1  "<omX>"
  Bus Selector/11 -> Mux4/3  "<omZ>"
  Bus Selector/2 -> [beta]  "<beta>"
  Merge1/1 -> qCmd/1
  PITCH_ATF/1(qCmdRad) -> Merge1/1
  PREV_FLCC_STATE/1 -> Bus Selector2/1
  Bus Selector/6 -> Mux3/2  "<pitch>"
  Mux3/1 -> [eulerAttiRad]
  Mux4/1 -> [pqrRad]
  tick/1 -> [tick]
  [eulerAttiRad] -> Demux1/1
  Demux1/1 -> PITCH_ATF/2(roll)
  Demux1/2 -> PITCH_ATF/3(pitch)
  [tick] -> PITCH_ATF/7(tick)
  PITCH_AGCAS_PARS/1(qCmdRad) -> Merge1/2
  Bus Selector/13 -> [ay]  "<accY>"
  [tick] -> PITCH_AGCAS_PARS/4(tick)
  ConfigureMPUG/1(maxPullUpG) -> [pullUpG]
  ConfigureMFPA/1(maxFlightPathAngle) -> [maxFPA]
  GCAWS/1 -> Bus Selector3/1
  Bus Selector3/1 -> ConfigureMPUG/1(pullUpGUint16)  "<pullUpGWrap>"
  Bus Selector3/2 -> ConfigureMFPA/1(maxFlightPathUint16)  "<maxFlightPathAngleWrap>"
  TF/1 -> Bus Selector4/1
  Bus Selector4/1 -> [gCmd]  "<verticalGCommand>"
  Merge2/1 -> OUT_recoveryStage/1
  Bus Selector/15 -> [velD]  "<velD>"
  [tick] -> If Action Subsystem/5(tick)
  [DYN_STATE] -> If Action Subsystem/3(DYN_STATE)
  [FLIGHT_CMD] -> If Action Subsystem/2(FLIGHT_CMD)
  [pitCtrlMode] -> If Action Subsystem/1(pitCtrlMode)
  pitDesDeg/1 -> If Action Subsystem/4(pitDesDeg)
  If Action Subsystem/2(OUT_recoveryStage) -> Merge2/3
  PITCH_AGCAS_PARS/2(OUT_recoveryStage) -> Merge2/2
  PITCH_ATF/2(OUT_recoveryStage) -> Merge2/1
  If Action Subsystem/1(qCmd) -> Merge1/3
  [DYN_STATE] -> PITCH_AGCAS_PARS/5(DYN_STATE)
  Bus Selector/8 -> [velX]  "<velX>"

== system M_FLCC/FlightController/AttitudeOuterLoop/Manual_LateralDirectional ==
  STICK : Inport
  DYN_STATE : Inport  Port=2
  Action Port : ActionPort  ActionPortLabel=if((u1== 0) | (u1 == 2))
  Manual_LatDir : MATLAB Function  TreatAsAtomicUnit=on
  pCmd : Outport
  rCmd : Outport  Port=2
  wires:
  STICK/1 -> Manual_LatDir/1(STICK)
  DYN_STATE/1 -> Manual_LatDir/2(DYN_STATE)
  Manual_LatDir/1(pCmd) -> pCmd/1
  Manual_LatDir/2(rCmd) -> rCmd/1

== system M_FLCC/FlightController/AttitudeOuterLoop/Manual_Longitudinal ==
  STICK : Inport
  DYN_STATE : Inport  Port=2
  Action Port : ActionPort  ActionPortLabel=if((u1== 0) | (u1 == 2))
  Constant_uint8_ : Constant  Value=0  OutDataTypeStr=uint8
  Manual_Long : MATLAB Function  TreatAsAtomicUnit=on
  qCmd : Outport
  OUT_recoveryStage : Outport  Port=2
  wires:
  Manual_Long/1(qCmd) -> qCmd/1
  DYN_STATE/1 -> Manual_Long/2(DYN_STATE)
  STICK/1 -> Manual_Long/1(STICK)
  Constant_uint8_/1 -> OUT_recoveryStage/1

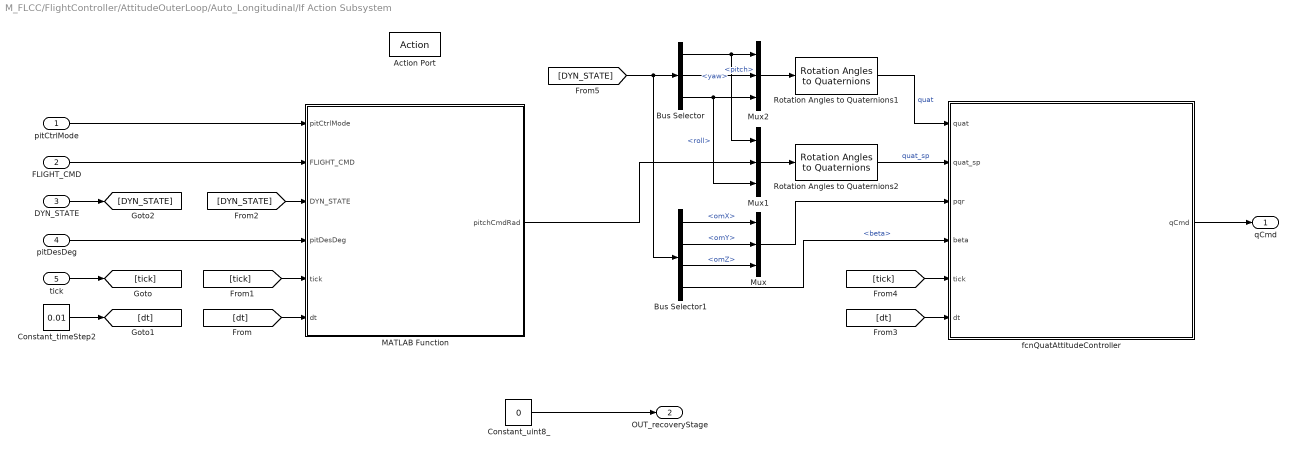
== system M_FLCC/FlightController/AttitudeOuterLoop/Auto_Longitudinal/If Action Subsystem ==
  pitCtrlMode : Inport
  FLIGHT_CMD : Inport  Port=2
  DYN_STATE : Inport  Port=3
  pitDesDeg : Inport  Port=4
  tick : Inport  Port=5
  Action Port : ActionPort  ActionPortLabel=else
  Bus Selector : BusSelector  OutputSignals=yaw,pitch,roll
  Bus Selector1 : BusSelector  OutputSignals=omX,omY,omZ,beta
  Constant_timeStep2 : Constant  Value=0.01
  Constant_uint8_ : Constant  Value=0  OutDataTypeStr=uint8
  MATLAB Function : MATLAB Function  TreatAsAtomicUnit=on
  Mux : Mux  Inputs=3
  Mux1 : Mux  Inputs=3
  Mux2 : Mux  Inputs=3
  Rotation Angles to Quaternions1 : sharedtransform/Rotation Angles to Quaternions  rotationOrder=ZYX  aMode=aMode
      settings: SourceProductBaseCode=AE,PW,DR,MT,VE
  Rotation Angles to Quaternions2 : sharedtransform/Rotation Angles to Quaternions  rotationOrder=ZYX  aMode=aMode
      settings: SourceProductBaseCode=AE,PW,DR,MT,VE
  fcnQuatAttitudeController : MATLAB Function  TreatAsAtomicUnit=on
  qCmd : Outport
  OUT_recoveryStage : Outport  Port=2
  wires:
  MATLAB Function/1(pitchCmdRad) -> Mux1/2
  pitCtrlMode/1 -> MATLAB Function/1(pitCtrlMode)
  FLIGHT_CMD/1 -> MATLAB Function/2(FLIGHT_CMD)
  pitDesDeg/1 -> MATLAB Function/4(pitDesDeg)
  Constant_uint8_/1 -> OUT_recoveryStage/1
  fcnQuatAttitudeController/1(qCmd) -> qCmd/1
  tick/1 -> [tick]
  Constant_timeStep2/1 -> [dt]
  [tick] -> MATLAB Function/5(tick)
  [dt] -> MATLAB Function/6(dt)
  DYN_STATE/1 -> [DYN_STATE]
  [DYN_STATE] -> MATLAB Function/3(DYN_STATE)
  [tick] -> fcnQuatAttitudeController/5(tick)
  [dt] -> fcnQuatAttitudeController/6(dt)
  Rotation Angles to Quaternions2/1 -> fcnQuatAttitudeController/2(quat_sp)  "quat_sp"
  [DYN_STATE] -> Bus Selector1/1, Bus Selector/1
  Rotation Angles to Quaternions1/1 -> fcnQuatAttitudeController/1(quat)  "quat"
  Bus Selector/1 -> Mux1/1, Mux2/1  "<yaw>"
  Bus Selector/2 -> Mux2/2  "<pitch>"
  Bus Selector/3 -> Mux1/3, Mux2/3  "<roll>"
  Mux2/1 -> Rotation Angles to Quaternions1/1
  Mux1/1 -> Rotation Angles to Quaternions2/1
  Bus Selector1/1 -> Mux/1  "<omX>"
  Bus Selector1/2 -> Mux/2  "<omY>"
  Bus Selector1/3 -> Mux/3  "<omZ>"
  Bus Selector1/4 -> fcnQuatAttitudeController/4(beta)  "<beta>"
  Mux/1 -> fcnQuatAttitudeController/3(pqr)

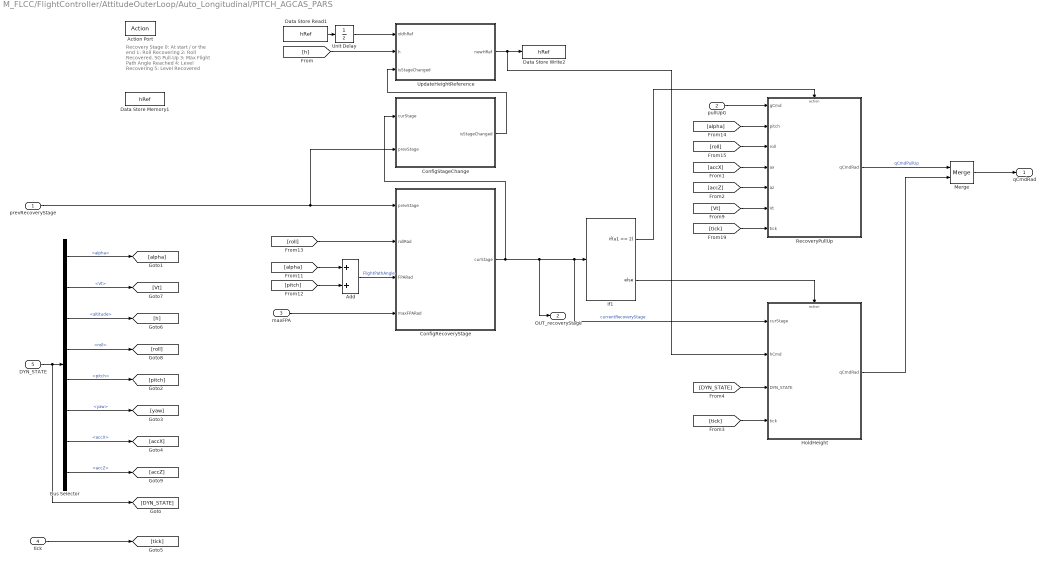
== system M_FLCC/FlightController/AttitudeOuterLoop/Auto_Longitudinal/PITCH_AGCAS_PARS ==
  note: Recovery Stage
      | 0: At start / or the end
      | 1: Roll Recovering
      | 2: Roll Recovered. 5G Pull-Up
      | 3: Max Flight Path Angle Reached
      | 4: Level Recovering
      | 5: Level Recovered
  prevRecoveryStage : Inport
  pullUpG : Inport  Port=2
  maxFPA : Inport  Port=3
  tick : Inport  Port=4
  DYN_STATE : Inport  Port=5
  Action Port : ActionPort  InitializeStates=reset  ActionPortLabel=elseif((u1 == 4) | (u1 == 5))
  Add : Sum
  Bus Selector : BusSelector  OutputSignals=alpha,Vt,altitude,roll,pitch,yaw,accX,accZ
  ConfigRecoveryStage : MATLAB Function  TreatAsAtomicUnit=on  SystemSampleTime=0.01
  ConfigStageChange : MATLAB Function  TreatAsAtomicUnit=on
  Data Store Memory1 : DataStoreMemory  DataStoreName=hRef  WriteAfterWriteMsg=warning  ShowAdditionalParam=off  OutDataTypeStr=double
      settings: LockScale=on
  Data Store Read1 : DataStoreRead  DataStoreName=hRef  IndexOptions=Index vector (dialog)  Indices=1  OutputSizes=1
  Data Store Write2 : DataStoreWrite  DataStoreName=hRef  IndexOptions=Index vector (dialog)  Indices=1  OutputSizes=1
  HoldHeight : Subsystem  TreatAsAtomicUnit=on
  If1 : If  IfExpression=u1 == 2
  Merge : Merge
  RecoveryPullUp : Subsystem  TreatAsAtomicUnit=on
  Unit Delay : UnitDelay  SampleTime=-1  HasFrameUpgradeWarning=on
  UpdateHeightReference : MATLAB Function  TreatAsAtomicUnit=on
  qCmdRad : Outport
  OUT_recoveryStage : Outport  Port=2
  wires:
  [accZ] -> RecoveryPullUp/5(az)
  [h] -> UpdateHeightReference/2(h)
  ConfigRecoveryStage/1(curStage) -> ConfigStageChange/1(curStage), OUT_recoveryStage/1, HoldHeight/1(curStage), If1/1  "currentRecoveryStage"
  prevRecoveryStage/1 -> ConfigStageChange/2(prevStage), ConfigRecoveryStage/1(prevStage)
  [roll] -> ConfigRecoveryStage/2(rollRad)
  [alpha] -> Add/1
  [pitch] -> Add/2
  UpdateHeightReference/1(newHRef) -> HoldHeight/2(hCmd), Data Store Write2/1
  Data Store Read1/1 -> Unit Delay/1
  Unit Delay/1 -> UpdateHeightReference/1(oldhRef)
  ConfigStageChange/1(isStageChanged) -> UpdateHeightReference/3(isStageChanged)
  If1/1 -> RecoveryPullUp/Action
  If1/2 -> HoldHeight/Action
  [Vt] -> RecoveryPullUp/6(Vt)
  maxFPA/1 -> ConfigRecoveryStage/4(maxFPARad)
  Add/1 -> ConfigRecoveryStage/3(FPARad)  "FlightPathAngle"
  pullUpG/1 -> RecoveryPullUp/1(gCmd)
  [alpha] -> RecoveryPullUp/2(pitch)
  [roll] -> RecoveryPullUp/3(roll)
  [accX] -> RecoveryPullUp/4(ax)
  Merge/1 -> qCmdRad/1
  RecoveryPullUp/1(qCmdRad) -> Merge/1  "qCmdPullUp"
  tick/1 -> [tick]
  [tick] -> RecoveryPullUp/7(tick)
  HoldHeight/1(qCmdRad) -> Merge/2
  [tick] -> HoldHeight/4(tick)
  DYN_STATE/1 -> [DYN_STATE], Bus Selector/1
  Bus Selector/1 -> [alpha]  "<alpha>"
  Bus Selector/2 -> [Vt]  "<Vt>"
  Bus Selector/3 -> [h]  "<altitude>"
  Bus Selector/4 -> [roll]  "<roll>"
  Bus Selector/5 -> [pitch]  "<pitch>"
  Bus Selector/6 -> [yaw]  "<yaw>"
  Bus Selector/7 -> [accX]  "<accX>"
  Bus Selector/8 -> [accZ]  "<accZ>"
  [DYN_STATE] -> HoldHeight/3(DYN_STATE)

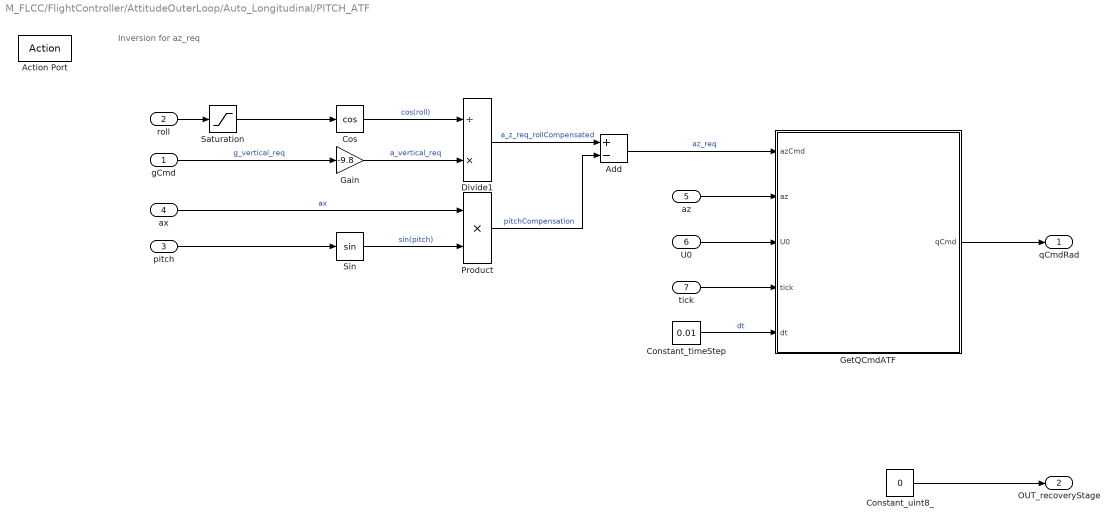
== system M_FLCC/FlightController/AttitudeOuterLoop/Auto_Longitudinal/PITCH_ATF ==
  note: Inversion for az_req
  gCmd : Inport
  roll : Inport  Port=2
  pitch : Inport  Port=3
  ax : Inport  Port=4
  az : Inport  Port=5
  U0 : Inport  Port=6
  tick : Inport  Port=7
  Action Port : ActionPort  ActionPortLabel=if((u1 == 3))
  Add : Sum  Inputs=+-
  Constant_timeStep : Constant  Value=0.01
  Constant_uint8_ : Constant  Value=0  OutDataTypeStr=uint8
  Cos : Trigonometry  Operator=cos
  Divide1 : Product  Inputs=/*
  Gain : Gain  Gain=-9.8
  GetQCmdATF : MATLAB Function  TreatAsAtomicUnit=on  SystemSampleTime=0.01
  Product : Product
  Saturation : Saturate  UpperLimit=85.0 * (pi/180)  LowerLimit=-85.0 * (pi/180)
  Sin : Trigonometry
  qCmdRad : Outport
  OUT_recoveryStage : Outport  Port=2
  wires:
  U0/1 -> GetQCmdATF/3(U0)
  gCmd/1 -> Gain/1  "g_vertical_req"
  Gain/1 -> Divide1/2  "a_vertical_req"
  Divide1/1 -> Add/1  "a_z_req_rollCompensated"
  Product/1 -> Add/2  "pitchCompensation"
  ax/1 -> Product/1  "ax"
  roll/1 -> Saturation/1
  pitch/1 -> Sin/1
  Sin/1 -> Product/2  "sin(pitch)"
  GetQCmdATF/1(qCmd) -> qCmdRad/1
  Constant_timeStep/1 -> GetQCmdATF/5(dt)  "dt"
  Cos/1 -> Divide1/1  "cos(roll)"
  Saturation/1 -> Cos/1
  Add/1 -> GetQCmdATF/1(azCmd)  "az_req"
  az/1 -> GetQCmdATF/2(az)
  tick/1 -> GetQCmdATF/4(tick)
  Constant_uint8_/1 -> OUT_recoveryStage/1

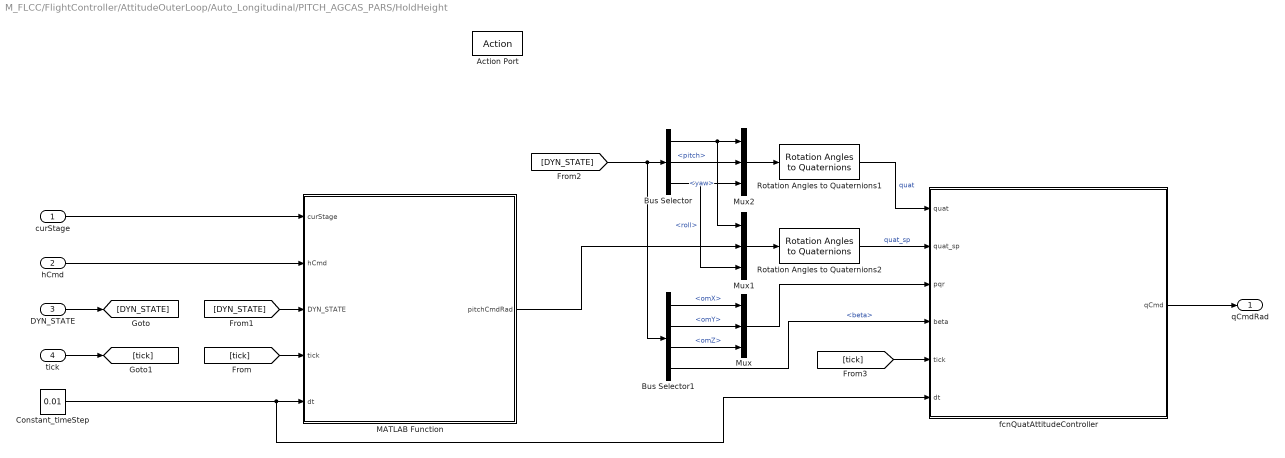
== system M_FLCC/FlightController/AttitudeOuterLoop/Auto_Longitudinal/PITCH_AGCAS_PARS/HoldHeight ==
  curStage : Inport
  hCmd : Inport  Port=2
  DYN_STATE : Inport  Port=3
  tick : Inport  Port=4
  Action Port : ActionPort  ActionPortLabel=else
  Bus Selector : BusSelector  OutputSignals=yaw,pitch,roll
  Bus Selector1 : BusSelector  OutputSignals=omX,omY,omZ,beta
  Constant_timeStep : Constant  Value=0.01
  MATLAB Function : MATLAB Function  TreatAsAtomicUnit=on
  Mux : Mux  Inputs=3
  Mux1 : Mux  Inputs=3
  Mux2 : Mux  Inputs=3
  Rotation Angles to Quaternions1 : sharedtransform/Rotation Angles to Quaternions  rotationOrder=ZYX  aMode=aMode
      settings: SourceProductBaseCode=AE,PW,DR,MT,VE
  Rotation Angles to Quaternions2 : sharedtransform/Rotation Angles to Quaternions  rotationOrder=ZYX  aMode=aMode
      settings: SourceProductBaseCode=AE,PW,DR,MT,VE
  fcnQuatAttitudeController : MATLAB Function  TreatAsAtomicUnit=on
  qCmdRad : Outport
  wires:
  Constant_timeStep/1 -> fcnQuatAttitudeController/6(dt), MATLAB Function/5(dt)
  Rotation Angles to Quaternions1/1 -> fcnQuatAttitudeController/1(quat)  "quat"
  MATLAB Function/1(pitchCmdRad) -> Mux1/2
  Bus Selector/2 -> Mux2/2  "<pitch>"
  Mux/1 -> fcnQuatAttitudeController/3(pqr)
  Bus Selector/3 -> Mux1/3, Mux2/3  "<roll>"
  Mux2/1 -> Rotation Angles to Quaternions1/1
  Bus Selector1/2 -> Mux/2  "<omY>"
  Bus Selector1/1 -> Mux/1  "<omX>"
  Bus Selector1/3 -> Mux/3  "<omZ>"
  [DYN_STATE] -> Bus Selector/1, Bus Selector1/1
  Mux1/1 -> Rotation Angles to Quaternions2/1
  Bus Selector/1 -> Mux1/1, Mux2/1  "<yaw>"
  Bus Selector1/4 -> fcnQuatAttitudeController/4(beta)  "<beta>"
  fcnQuatAttitudeController/1(qCmd) -> qCmdRad/1
  hCmd/1 -> MATLAB Function/2(hCmd)
  curStage/1 -> MATLAB Function/1(curStage)
  [tick] -> MATLAB Function/4(tick)
  tick/1 -> [tick]
  DYN_STATE/1 -> [DYN_STATE]
  [DYN_STATE] -> MATLAB Function/3(DYN_STATE)
  Rotation Angles to Quaternions2/1 -> fcnQuatAttitudeController/2(quat_sp)  "quat_sp"
  [tick] -> fcnQuatAttitudeController/5(tick)

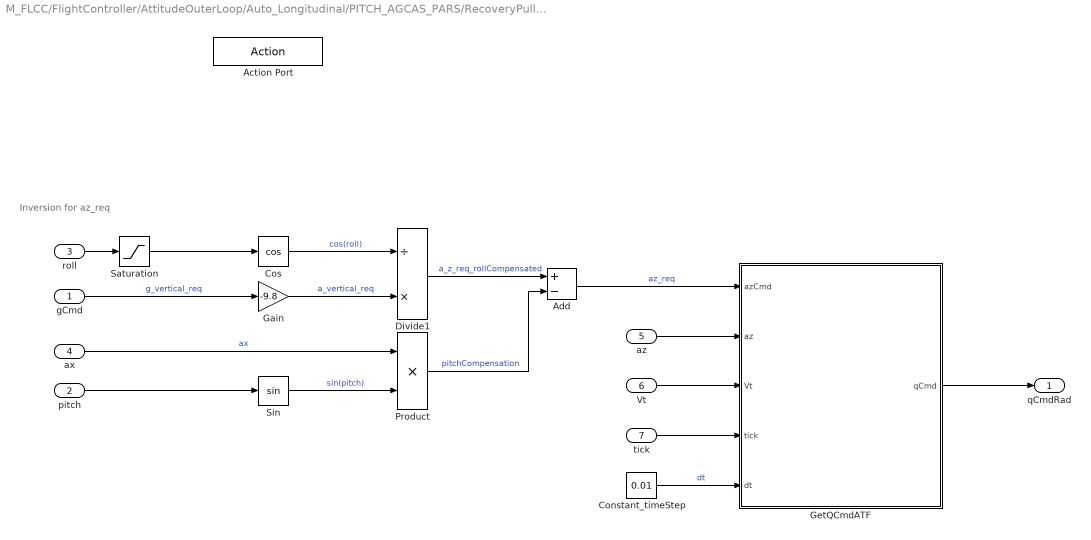
== system M_FLCC/FlightController/AttitudeOuterLoop/Auto_Longitudinal/PITCH_AGCAS_PARS/RecoveryPullUp ==
  note: Inversion for az_req
  gCmd : Inport
  pitch : Inport  Port=2
  roll : Inport  Port=3
  ax : Inport  Port=4
  az : Inport  Port=5
  Vt : Inport  Port=6
  tick : Inport  Port=7
  Action Port : ActionPort  ActionPortLabel=if(u1 == 2)
  Add : Sum  Inputs=+-
  Constant_timeStep : Constant  Value=0.01
  Cos : Trigonometry  Operator=cos
  Divide1 : Product  Inputs=/*
  Gain : Gain  Gain=-9.8
  GetQCmdATF : MATLAB Function  TreatAsAtomicUnit=on  SystemSampleTime=0.01
  Product : Product
  Saturation : Saturate  UpperLimit=85.0 * (pi/180)  LowerLimit=-85.0 * (pi/180)
  Sin : Trigonometry
  qCmdRad : Outport
  wires:
  az/1 -> GetQCmdATF/2(az)
  Constant_timeStep/1 -> GetQCmdATF/5(dt)  "dt"
  Divide1/1 -> Add/1  "a_z_req_rollCompensated"
  ax/1 -> Product/1  "ax"
  tick/1 -> GetQCmdATF/4(tick)
  Product/1 -> Add/2  "pitchCompensation"
  Cos/1 -> Divide1/1  "cos(roll)"
  GetQCmdATF/1(qCmd) -> qCmdRad/1
  Gain/1 -> Divide1/2  "a_vertical_req"
  Saturation/1 -> Cos/1
  Add/1 -> GetQCmdATF/1(azCmd)  "az_req"
  gCmd/1 -> Gain/1  "g_vertical_req"
  Sin/1 -> Product/2  "sin(pitch)"
  Vt/1 -> GetQCmdATF/3(Vt)
  pitch/1 -> Sin/1
  roll/1 -> Saturation/1

== matlab function M_FLCC/FlightController/AttitudeOuterLoop/Auto_Longitudinal/If Action Subsystem/fcnQuatAttitudeController ==
  data: quat input; qCmd output; quat_sp input; pqr input; beta input; tick input; dt input
function qCmd = fcnQuatAttitudeController(quat, quat_sp, pqr, beta, tick, dt)
%fcnQuatAttitudeController
%
% -- Input --
% quat : quaternion vector (1-by-4 column vector of real numbers)
% quat_sp : (set point) quaternion vector (1-by-4 column vector of real numbers)
% -- Output --
% pqrCmd : angular rate command (3-by-1 column vector of real numbers)

persistent firstRun prev_quat_err prevTick
if isempty(prev_quat_err)
    prev_quat_err = [1, 0, 0, 0];
end
if isempty(firstRun)
    firstRun = true;
end
if isempty(prevTick)
    prevTick = uint32(0);
end

% Initialize Integral control term
if (tick - prevTick ) >= uint32(2)
    prev_quat_err = [1, 0, 0, 0];
end

% Intialize
qCmd = 0.0;
quat_err = zeros(1,4);
eul_ypr = zeros(1,3);
rol = 0.0;
pit = 0.0;

% Controller gain
Kp_p = 2.0;
Kp_q = 0.2;
Kd_q = -0.01;
% Kd_q = -0.0;
Kp_r = 0.0;
Kp_beta = -0.03;
D2R = pi/180;

% Attitude error quaternion
quat_err = quatmultiply( quatconj(quat'), quat_sp' );
quat_err = quatnormalize(quat_err);

% Convert a quat_err to axis-angle representation
ang_err = 2 * acos(quat_err(1));
if ( (IsNear(quat_err(1), 1)) || (IsNear(quat_err(1), -1)) )
    u_x = 0.0;
    u_y = 0.0;
    u_z = 0.0;
else
    u_x = quat_err(2) / sqrt(1 - quat_err(1)^2);
    u_y = quat_err(3) / sqrt(1 - quat_err(1)^2);
    u_z = quat_err(4) / sqrt(1 - quat_err(1)^2);
end

% % Choose a shorter rotation ang_err
if (ang_err > pi)
    ang_err = abs(ang_err - 2*pi);
    u_x = -u_x;
    u_y = -u_y;
    u_z = -u_z;
else
end

% Convert the new attitude error from the axis-angle representation back
% to quaternion form
quat_err(1) = cos(ang_err/2);
quat_err(2) = u_x * sin(ang_err/2);
quat_err(3) = u_y * sin(ang_err/2);
quat_err(4) = u_z * sin(ang_err/2);

eul_ypr = quat2eul(quat', 'ZYX');
% % Ensure we have shorter rotation
if (quat_err(1) < 0)
    quat_err(1) = -quat_err(1);
    quat_err(2) = -quat_err(2);
    quat_err(3) = -quat_err(3);
    quat_err(4) = -quat_err(4);
else
end

% Normalize 
quat_err = quatnormalize(quat_err);

% Euler angles from quaternion
eul_ypr = quat2eul(quat', 'ZYX');
rol = eul_ypr(3);
pit = eul_ypr(2);

% Inversion from attitude kinematics
q = pqr(2);
r = pqr(3);

if abs(pit) > 80*D2R
    pTrim = 0;
    qTrim = 0;
else
    pTrim  =  (- (q * sin(rol) * tan(pit)) - (r * cos(rol) * tan(pit)));
    qTrim  =  (   r * tan(rol));
end
% rTrim  =  (   qTrim / tan(phi));
rTrim  = 0;

% Calculate angular rate command
if (firstRun)
    DTerm = [1, 0, 0, 0];
else
    DTerm = (quat_err - prev_quat_err)/dt;
    DTerm(3) = fcnSaturation(DTerm(3), 0.1);
end
pCmd = pTrim + 2 * Kp_p * quat_err(2);
qCmd = qTrim + 2 * Kp_q * quat_err(3) + Kd_q * DTerm(3);
rCmd = rTrim + 2 * Kp_r * quat_err(4) + Kp_beta * (0 - beta);
% pCmd = K_p * quat_err(2);
% qCmd = K_q * quat_err(3);
% rCmd = rTrim + 2 * K_r * quat_err(4) + Kbeta * (0 - beta);


% Saturate command
plim = 25 * D2R;
qlim = 25 * D2R;
rlim = 20 * D2R;

pCmd = fcnSaturation(pCmd, plim);
qCmd = fcnSaturation(qCmd, qlim);
rCmd = fcnSaturation(rCmd, rlim);

% Output
pqrCmd = [pCmd; qCmd; rCmd];

firstRun = false;
prev_quat_err = quat_err;
prevTick = tick;
end


function in = fcnSaturation(in, lim)

if abs(in)>lim
    in = lim*sign(in);
end

end

== matlab function M_FLCC/FlightController/GroundModeManager ==
  data: DYN_STATE input Bus: BUS_DYN_STATE; PREV_FLCC_STATE input Bus: BUS_FLCC_AP_STATE; inFlying output; groundStage output; tick input; h0 output
function [inFlying, groundStage, h0] = GroundModeManager(DYN_STATE, PREV_FLCC_STATE, tick)
%GroundModeManager 현재 항공기가 지상운동중인지, 비행중인지를 식별하고
% 지상운동일 경우 이륙절차 스케쥴링을 진행한다.
% --- INPUT ---
% DTN_STATE: 현재 항공기 상태 bus object(BUS_DYN_STATE)
% PREV_FLCC_STATE: 이전 실행에서의 bus object(BUS_FLCC_AP_STATE)
% tick: 현재 실행에서의 FLCC 모델의 작동 tick이자 호출 횟수 (uint32)
% --- OUTPUT ---
% inFlying: 비행중 플래그 (true: 비행중/ false: 지상)
% groundStage: 
%               [0 = JUST BOOTED UP]
%               [1 = GROUND IDLE]
%               [2 = TAXING]
%               [3 = READY TAKEOFF]
%               [4 = GROUND ROLL]
%               [5 = ROTATION]
%               [6 = TO AIR TRANSITION]
%               [7 = CLIMBOUT]
%               [8 = IN FLYING]
%               [9 = CRASHES]
% h0:
% -------------------------------------------------------------------------
persistent mem_groundStage tickCountTO tickCountCO
if isempty(mem_groundStage)
    mem_groundStage = uint8(0);
end
if isempty(tickCountTO)
    tickCountTO = uint32(0);
end
if isempty(tickCountCO)
    tickCountCO = uint32(0);
end
h0 = PREV_FLCC_STATE.h0;

% Initialize
inFlying = PREV_FLCC_STATE.inFlying;
groundStage = PREV_FLCC_STATE.groundStage;

% CONSTANTS
KTS2MPS = 0.51444444444;
DEG2RAD = pi/180;

Vt_TO = 170 * KTS2MPS;
pitch_TO = 15 * DEG2RAD;

% Rearrange
pitch = DYN_STATE.pitch;
alt = DYN_STATE.altitude;

Vt = sqrt( DYN_STATE.velN^2 + DYN_STATE.velE^2 + DYN_STATE.velD^2 );


%% STATE MACHINE

% Configure [ IN FLYING ] or [ ON GROUND ]
if (PREV_FLCC_STATE.inFlying)
    if ( alt < h0 - 5.0 )
        inFlying = false;
        groundStage = uint8(9);
    else
        inFlying = true;
        groundStage = PREV_FLCC_STATE.groundStage;
        return
    end
else % ON_GROUND
    if ( (Vt > Vt_TO + 20) && (alt > h0 + 100) )
        inFlying = true;
        groundStage = uint8(8);
        return
    else
        inFlying = false;
    end
end

% Configure ground stage [ ON GROUND ]
switch PREV_FLCC_STATE.groundStage
    case uint8(0) % Just booted up
        groundStage = uint8(1);
    case uint8(1) % Ground idle
        if Vt > 5.0
            groundStage = uint8(2);
        elseif tick > uint32(2000)
            groundStage = uint8(2);
        end
    case uint8(2) % Taxing
        if Vt < 1.0
            groundStage = uint8(3);
        elseif tick > uint32(15000)
            groundStage = uint8(3);
        end
    case uint8(3) % Ready to take-off
        tickCountTO = tickCountTO + uint32(1);
        if tickCountTO > uint32(3000)
            groundStage = uint8(4);
            tickCountTO = uint32(0);
        elseif (Vt > 20.0)
            groundStage = uint8(4);
            tickCountTO = uint32(0);
        end
    case uint8(4) % Ground roll
        if (Vt > Vt_TO)
            groundStage = uint8(5);
        end
    case uint8(5) % Rotation
        if (pitch > 0.75 * pitch_TO)
            groundStage = uint8(6);
        end
    case uint8(6) % To air transition
        if (alt > h0 + 50)
            groundStage = uint8(7);
        end
    case uint8(7) % Climb out
        tickCountCO = tickCountCO + uint32(1);
        if tickCountCO > uint32(500)
            groundStage = uint8(8);
            tickCountCO = uint32(0);
        end
    otherwise

end

entryAlarmMessage(groundStage, tick);
% Memory
mem_groundStage = PREV_FLCC_STATE.groundStage;

 
end


function entryAlarmMessage(groundStage, tick)
persistent prevGroundStage
if isempty(prevGroundStage)
    prevGroundStage = uint8(0);
end

if (prevGroundStage ~= groundStage)
    switch groundStage
        case uint8(0)
            fprintf("Just Booted Up [tick: %u]\r\n", tick);
        case uint8(1)
            fprintf("Ground Idle [tick: %u]\r\n", tick);
        case uint8(2)
            fprintf("Taxing [tick: %u]\r\n", tick);
        case uint8(3)
            fprintf("Ready To Take-Off [tick: %u]\r\n", tick);
        case uint8(4)
            fprintf("Ground Roll [tick: %u]\r\n", tick);
        case uint8(5)
            fprintf("Rotation [tick: %u]\r\n", tick);
        case uint8(6)
            fprintf("To Air Transition [tick: %u]\r\n", tick);
        case uint8(7)
            fprintf("Climb Out [tick: %u]\r\n", tick);
        case uint8(9)
            fprintf("Crashed [tick: %u]\r\n", tick);
        otherwise

    end
else
end

prevGroundStage = groundStage;

end

== matlab function M_FLCC/FlightController/TickCounter ==
  data: PREV_FLCC_STATE input; tick output
function tick = TickCounter(PREV_FLCC_STATE)
%TickCounter FLCC 모델의 작동 tick을 갱신한다
% --- INPUT ---
% PREV_FLCC_STATE: 이전 실행에서의 bus object(BUS_FLCC_AP_STATE)
% --- OUTPUT ---
% tick: 현재 실행에서의 FLCC 모델의 작동 tick이자 호출 횟수 (uint32)
% -------------------------------------------------------------------------

if (PREV_FLCC_STATE.tick == uint32(4294967295))
    tick = uint32(0);
else
    tick = PREV_FLCC_STATE.tick + uint32(1);
end

== matlab function M_FLCC/InitNUpdateMapCache/UpdateCache/UpdateCache ==
  data: result output; lat input; lon input; hDEM output
function [result, hDEM] = UpdateCache(lat, lon)
%UpdateCache

% Persistent variables
persistent latPrev lonPrev
if isempty(latPrev)
    latPrev = 0.0;
end
if isempty(lonPrev)
    lonPrev = 0.0;
end

hDEM = 0.0;

% Initialize output
result = int32(1);

if ( abs(lat - latPrev) > 0.05 ) || ( abs(lon - lonPrev) > 0.05)
    result = coder.ceval('UpdateCache', lat, lon);
    hDEM = coder.ceval('MAPGetTerrainHeight', lat, lon);

    if result == 0
        latPrev = lat;
        lonPrev = lon;
    end
else
    
end

== matlab function M_FLCC/FlightController/AttitudeOuterLoop/Auto_Longitudinal/PITCH_AGCAS_PARS/HoldHeight/MATLAB Function ==
  data: curStage input; pitchCmdRad output; hCmd input; DYN_STATE input; tick input; dt input
function pitchCmdRad = shapePitchCmd(curStage, hCmd, DYN_STATE, tick, dt)
%shapePitchCmd
% --- INPUT ---
% pitCtrlMode : [0=OFF] [1=ATT HOLD] [2=ALT HOLD] [3=ATF] 
%               [4=AGCAS] [5=PARS] uint8
% [FLIGHT_CMD]
% .nextAlt : desired altitude [m]
% [DYN_STATE]
% .Vt : current vehicle's total airspeed [deg]
% .beta : sideslip angle
% .alt
% .alpha
% .eulerAtti
% pitDesDeg : desired ptich angle in ATT HOLD mode
% --- Output ---
% pitchCmdRad : pitch command [rad]

persistent hErrInt prevTick hDotInt
if isempty(hErrInt)
    hErrInt = 0.0; 
end
if isempty(prevTick)
    prevTick = uint32(0);
end
if isempty(hDotInt)
    hDotInt = 0.0;
end

% Initialize
pitchCmdRad = 0.0;

% Constant
D2R = pi/180;

% Rearrange
alpha = DYN_STATE.alpha;
Vt = DYN_STATE.Vt;
h = DYN_STATE.altitude;
pitch = DYN_STATE.pitch;
hDot = -DYN_STATE.velD;

switch curStage
    case uint8(3)
        %% Altitude Hold
        % PI Control gains for altitude controller
        Kh_p = 0.25;
        Kh_i = 0.01;
        KhDot_p = 4.5;
        KhDot_i = 0.5;

        % Initialize Integral control term when switched
        if (tick - prevTick ) >= uint32(2)
            hErrInt = 0.0;
            hDotInt = 0.0;
        end

        % Control error term & limitation
        hLim    = 100;
        hErrLim = 20;
        hDotlim = 30;
        pitLim  = 20*D2R;
        
        hErr    = fcnSaturation(hCmd - h, hLim);
        hErrInt = fcnSaturation(hErrInt + hErr*dt, hErrLim);

        hDotCmd = fcnSaturation(Kh_p*hErr + Kh_i*hErrInt, hDotlim);
        hDotInt = fcnSaturation(hDotInt + (hDotCmd - hDot)*dt, 10);

        if abs(Vt*cos(pitch)) > 10
            gamCmd = (KhDot_p * (hDotCmd - hDot) + KhDot_i * hDotInt) ...
                / (Vt*cos(pitch));
        else
            gamCmd = (KhDot_p * (hDotCmd - hDot) + KhDot_i * hDotInt);
        end

        % Pitch command
        pitchCmdRad  = fcnSaturation(gamCmd + alpha, pitLim);
        
        % Update Tick
        prevTick = tick;
            
    otherwise
        %% Default
        pitchCmdRad = pitch;
end

end

%%
function in = fcnSaturation(in, lim)
    if abs(in) > lim
        in = lim*sign(in);
    end
end
